simulink model "symbolTask"  (R2012b)
settings: Solver=FixedStepDiscrete  StartTime=0.0  StopTime=10.0  FixedStep=0.001  RelTol=1e-3
undefined symbols (not defined in the file): acquireMethods, autoplayMovementDuration, autoplayReactionTime, autoplayRotationDuration, autoplayRotationStart, centerOffset, clickPercentage, clickRefractoryPeriod, clickTargetColor, clickTargetHoverColor, cuedText, cuedTextLength, cumulativeDwell, cursorColorClick, cursorColorClosed, cursorColorOpen, cursorDiameter, cursorNeuralColor, cursorNonneuralColor, delayOrder, delayPeriodGainScale, displayObject, doHeadSpeedFail, drawNumbersOnTargets, dwellRefractoryPeriod, errorAssistAxis, errorAssistR, errorAssistTheta, expRandBinSize, expRandMax, expRandMin, expRandMu, eyeMode, failOnLiftoff, failurePenalty, falseClickFails, fingerPositionTolerance, fixedSeqMode, freePlayMode, gain, gloveBias, gloveLPDenominator, gloveLPNumerator, gloveNonlinearCorrection, gloveXCorrection, gloveYCorrection, gridEdges, gridTilesEachDim, headSpeedCap, holdDuration, holdTime, initialInput, initialLockout, initialState, inputType, keyboard, keyboardDims, keyPressedTime, lockFingerPosition, maxTaskTime ... (+103)
settings Model: Creator=gilja  LastModifiedBy=NPTL
settings SolverCC: EnableConcurrentExecution=on  ConcurrentTasks=on
settings DataIOCC: SaveOutput=off  SignalLogging=off  SaveTime=off
settings OptimizationCC: InlineParams=on  InlineInvariantSignals=on  EnhancedBackFolding=on  EfficientFloat2IntCast=on  SimCompilerOptimization=On
settings DebuggingCC: UnderspecifiedInitializationDetection=Simplified
settings HardwareCC: ProdIntDivRoundTo=Zero  ProdEndianess=LittleEndian  ProdHWDeviceType=Generic->32-bit x86 compatible
settings RTWCC: SystemTargetFile=xpctarget.tlc  TemplateMakefile=xpc_default_tmf  Description=xPC Target  ProcessScript=xpctarget_make_rtw_hook  RTWCompilerOptimization=On
settings CodeAppCC: MaxIdLength=62
settings xpcTargetCC: TargetFcnLib=ansi_tfl_table_tmw.mat  CodeReplacementLibrary=XPC_BLAS  ParMdlRefBuildCompliant=on  ConcurrentExecutionCompliant=on  CombineSignalStateStructs=off  GRTInterface=on  xPCTaskExecutionProfile=on  xPCRL32EventNumber=5000  xPCisDownloadable=off  xPCLoadParamSetFile=off  xPCConcurrentTasks=off  xPCEnableSFAnimation=off

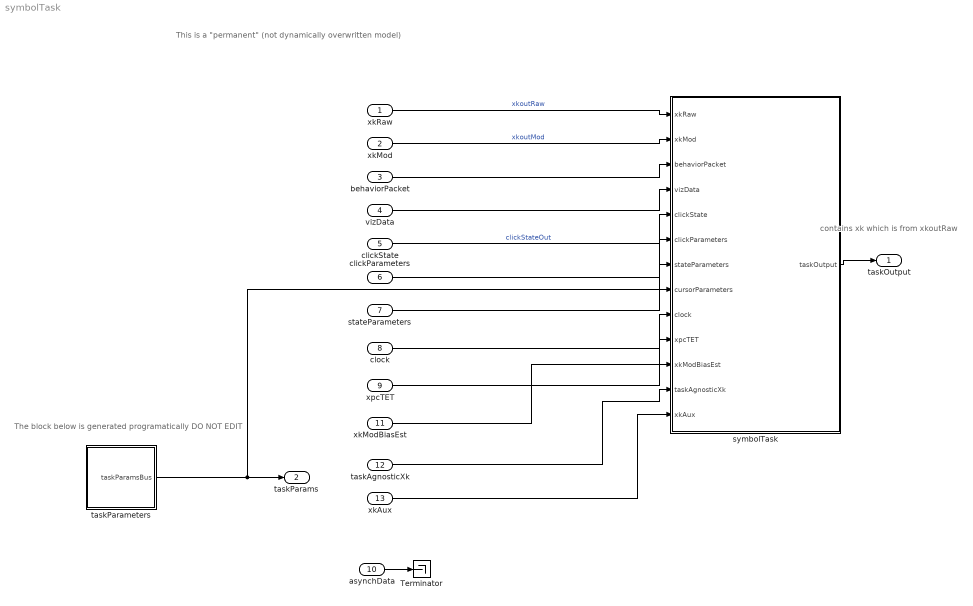
== system symbolTask ==
  note: contains xk which is
      | from xkoutRaw
  note: This is a "permanent" (not dynamically overwritten model)
  note: The block below is generated programatically
      | DO NOT EDIT
  xkRaw : Inport  OutDataTypeStr=double  PortDimensions=[double(xkConstants.NUM_STATE_DIMENSIONS),1]  SampleTime=[0.001,0]
  xkMod : Inport  Port=2  OutDataTypeStr=double  PortDimensions=[double(xkConstants.NUM_STATE_DIMENSIONS),1]  SampleTime=[0.001,0]
  behaviorPacket : Inport  Port=3  OutDataTypeStr=Bus: behaviorPacketBus  SampleTime=[0.001,0]
  vizData : Inport  Port=4  OutDataTypeStr=Bus: peripheralData  SampleTime=[0.001,0]
  clickState : Inport  Port=5  OutDataTypeStr=uint16  PortDimensions=1  SampleTime=[0.001,0]
  clickParameters : Inport  Port=6  OutDataTypeStr=Bus: clickParametersBus  SampleTime=[0.001,0]
  stateParameters : Inport  Port=7  OutDataTypeStr=Bus: stateParams  SampleTime=[0.001,0]
  clock : Inport  Port=8  OutDataTypeStr=uint32  PortDimensions=1  SampleTime=[0.001,0]
  xpcTET : Inport  Port=9  OutDataTypeStr=double  PortDimensions=1  SampleTime=[0.001,0]
  asynchData : Inport  Port=10  OutDataTypeStr=Bus: peripheralData  SampleTime=[0.001,0]
  xkModBiasEst : Inport  Port=11  OutDataTypeStr=double  PortDimensions=[double(xkConstants.NUM_STATE_DIMENSIONS),1]  SampleTime=[0.001,0]
  taskAgnosticXk : Inport  Port=12  OutDataTypeStr=double  PortDimensions=[double(xkConstants.NUM_STATE_DIMENSIONS),1]  SampleTime=[0.001,0]
  xkAux : Inport  Port=13  OutDataTypeStr=double  PortDimensions=[double(xkConstants.NUM_STATE_DIMENSIONS),1]  SampleTime=[0.001,0]
  Terminator : Terminator
  symbolTask : MATLAB Function  TreatAsAtomicUnit=on
  taskParameters : Subsystem
  taskOutput : Outport  OutDataTypeStr=Bus: taskOutput  PortDimensions=1  SampleTime=[0.001,0]  BusOutputAsStruct=on
  taskParams : Outport  Port=2  OutDataTypeStr=Bus: taskParamsBus  SampleTime=[0.001,0]
  wires:
  xkRaw/1 -> symbolTask/1(xkRaw)  "xkoutRaw"
  behaviorPacket/1 -> symbolTask/3(behaviorPacket)
  vizData/1 -> symbolTask/4(vizData)
  clickState/1 -> symbolTask/5(clickState)  "clickStateOut"
  clickParameters/1 -> symbolTask/6(clickParameters)
  clock/1 -> symbolTask/9(clock)
  xpcTET/1 -> symbolTask/10(xpcTET)
  stateParameters/1 -> symbolTask/7(stateParameters)
  taskParameters/1(taskParamsBus) -> taskParams/1, symbolTask/8(cursorParameters)
  symbolTask/1(taskOutput) -> taskOutput/1
  asynchData/1 -> Terminator/1
  xkMod/1 -> symbolTask/2(xkMod)  "xkoutMod"
  xkModBiasEst/1 -> symbolTask/11(xkModBiasEst)
  taskAgnosticXk/1 -> symbolTask/12(taskAgnosticXk)
  xkAux/1 -> symbolTask/13(xkAux)

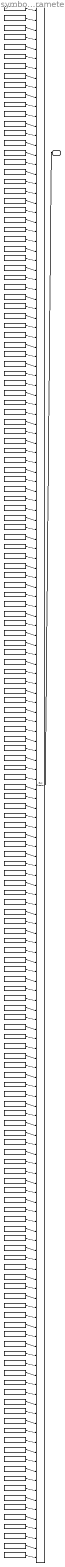
== system symbolTask/taskParameters ==
  BusOutput : BusCreator  Inputs=targetDiameter,maxTaskTime,holdTime,trialTimeout,numTrials,randomSeed,expRandMu,expRandMin,expRandMax,expRandBinSize,taskType,targetInds,numTargets,gain,failurePenalty,cursorDiameter,inputType,gloveBias,useRandomDelay,mouseOffset,workspaceX,workspaceY,workspaceZ,workspaceR,workspaceR2,showScores,trialsPerScore,cursorColorClick,recenterOnFail,recenterOnSuccess,recenterDelay,initialInput,clickPercentage,lockFingerPosition,fingerPositionTolerance,failOnLiftoff,errorAssistR,errorAssistTheta,errorAssistAxis,useGloveLPF,gloveLPNumerator,gloveLPDenominator,gloveNonlinearCorrection,gloveYCorrection,gloveXCorrection,useMouseLPF,soundOnFail,soundOnGo,soundOnSuccess,soundOnOverTarget,mouseLPNumerator,mouseLPDenominator,stopOffTarget,stopOnClick,outputType,xk2HorizontalPos,xk2HorizontalVel,xk2VerticalPos,xk2VerticalVel,xk2DepthPos,xk2DepthVel,xk2RotatePos,xk2RotateVel,xk2Rotate2Pos,xk2Rotate2Vel,gridEdges,gridTilesEachDim,selectionRefractoryMS,autoplayReactionTime,autoplayMovementDuration,powerGain,powerGainUnityCrossing,targetRotDiameter,autoplayRotationStart,autoplayRotationDuration,randomTaskTargetDiameters,randomTaskTargetRotDiameters,randomTaskBoundaries,numDisplayDims,cursorColorOpen,cursorColorClosed,showXYZaura,displayObject,preTrialLength,targetDiameters,numTargetDiameters,minTargetDistance,targetDelay,targetSpaceX,targetSpaceY,clickTargetColor,clickTargetHoverColor,falseClickFails,splitDimensions,vmrTheta,doHeadSpeedFail,headSpeedCap,eyeMode,speedTaskMode,delayPeriodGainScale,wiaMode,showWiaText,freePlayMode,drawNumbersOnTargets,xkRawSpeedCap,movementDuration,holdDuration,restDuration,returnDuration,repsPerBlock,whichMovements,movementOrder,delayOrder,clickRefractoryPeriod,xpcVelocityOutputPeriodMS,outputVelocityScaling,screenUpdateRate,targetDevice,playSpokenCues,numTargetsInSeq,targetSeq,seqReadyTime,seqRehearseTime,rotateSeqCues,numRepsPerSeq,rehearsalOrder,rehearsalTimes,pathMode,memorizeMode,fixedSeqMode,sequenceMatrix,keyboard,resetDisplay,cursorNeuralColor,cursorNonneuralColor,centerOffset,scoreTime,cuedTextLength,cuedText,keyboardDims,recenterFullscreen,soundOnError,acquireMethods,cumulativeDwell,showBackspace,showStartStop,showTargetText,showTypedText,showCueOnTarget,showCueOffTarget,recenterOffset,dwellRefractoryPeriod,keyPressedTime,initialLockout,initialState,symbolMoveTimeOne,symbolRehearseTime,symbolGetReadyTime,symbolMoveTimeTwo,symbolVMRMode,symbolVMRRot,pc1MouseInControlMode  OutDataTypeStr=Bus: taskParamsBus
  acquireMethods : Constant  Value=acquireMethods
  autoplayMovementDuration : Constant  Value=autoplayMovementDuration
  autoplayReactionTime : Constant  Value=autoplayReactionTime
  autoplayRotationDuration : Constant  Value=autoplayRotationDuration
  autoplayRotationStart : Constant  Value=autoplayRotationStart
  centerOffset : Constant  Value=centerOffset
  clickPercentage : Constant  Value=clickPercentage
  clickRefractoryPeriod : Constant  Value=clickRefractoryPeriod
  clickTargetColor : Constant  Value=clickTargetColor
  clickTargetHoverColor : Constant  Value=clickTargetHoverColor
  cuedText : Constant  Value=cuedText
  cuedTextLength : Constant  Value=cuedTextLength
  cumulativeDwell : Constant  Value=cumulativeDwell
  cursorColorClick : Constant  Value=cursorColorClick
  cursorColorClosed : Constant  Value=cursorColorClosed
  cursorColorOpen : Constant  Value=cursorColorOpen
  cursorDiameter : Constant  Value=cursorDiameter
  cursorNeuralColor : Constant  Value=cursorNeuralColor
  cursorNonneuralColor : Constant  Value=cursorNonneuralColor
  delayOrder : Constant  Value=delayOrder
  delayPeriodGainScale : Constant  Value=delayPeriodGainScale
  displayObject : Constant  Value=displayObject
  doHeadSpeedFail : Constant  Value=doHeadSpeedFail
  drawNumbersOnTargets : Constant  Value=drawNumbersOnTargets
  dwellRefractoryPeriod : Constant  Value=dwellRefractoryPeriod
  errorAssistAxis : Constant  Value=errorAssistAxis
  errorAssistR : Constant  Value=errorAssistR
  errorAssistTheta : Constant  Value=errorAssistTheta
  expRandBinSize : Constant  Value=expRandBinSize
  expRandMax : Constant  Value=expRandMax
  expRandMin : Constant  Value=expRandMin
  expRandMu : Constant  Value=expRandMu
  eyeMode : Constant  Value=eyeMode
  failOnLiftoff : Constant  Value=failOnLiftoff
  failurePenalty : Constant  Value=failurePenalty
  falseClickFails : Constant  Value=falseClickFails
  fingerPositionTolerance : Constant  Value=fingerPositionTolerance
  fixedSeqMode : Constant  Value=fixedSeqMode
  freePlayMode : Constant  Value=freePlayMode
  gain : Constant  Value=gain
  gloveBias : Constant  Value=gloveBias
  gloveLPDenominator : Constant  Value=gloveLPDenominator
  gloveLPNumerator : Constant  Value=gloveLPNumerator
  gloveNonlinearCorrection : Constant  Value=gloveNonlinearCorrection
  gloveXCorrection : Constant  Value=gloveXCorrection
  gloveYCorrection : Constant  Value=gloveYCorrection
  gridEdges : Constant  Value=gridEdges
  gridTilesEachDim : Constant  Value=gridTilesEachDim
  headSpeedCap : Constant  Value=headSpeedCap
  holdDuration : Constant  Value=holdDuration
  holdTime : Constant  Value=holdTime
  initialInput : Constant  Value=initialInput
  initialLockout : Constant  Value=initialLockout
  initialState : Constant  Value=initialState
  inputType : Constant  Value=inputType
  keyPressedTime : Constant  Value=keyPressedTime
  keyboard : Constant  Value=keyboard
  keyboardDims : Constant  Value=keyboardDims
  lockFingerPosition : Constant  Value=lockFingerPosition
  maxTaskTime : Constant  Value=maxTaskTime
  memorizeMode : Constant  Value=memorizeMode
  minTargetDistance : Constant  Value=minTargetDistance
  mouseLPDenominator : Constant  Value=mouseLPDenominator
  mouseLPNumerator : Constant  Value=mouseLPNumerator
  mouseOffset : Constant  Value=mouseOffset
  movementDuration : Constant  Value=movementDuration
  movementOrder : Constant  Value=movementOrder
  numDisplayDims : Constant  Value=numDisplayDims
  numRepsPerSeq : Constant  Value=numRepsPerSeq
  numTargetDiameters : Constant  Value=numTargetDiameters
  numTargets : Constant  Value=numTargets
  numTargetsInSeq : Constant  Value=numTargetsInSeq
  numTrials : Constant  Value=numTrials
  outputType : Constant  Value=outputType
  outputVelocityScaling : Constant  Value=outputVelocityScaling
  pathMode : Constant  Value=pathMode
  pc1MouseInControlMode : Constant  Value=pc1MouseInControlMode
  playSpokenCues : Constant  Value=playSpokenCues
  powerGain : Constant  Value=powerGain
  powerGainUnityCrossing : Constant  Value=powerGainUnityCrossing
  preTrialLength : Constant  Value=preTrialLength
  randomSeed : Constant  Value=randomSeed
  randomTaskBoundaries : Constant  Value=randomTaskBoundaries
  randomTaskTargetDiameters : Constant  Value=randomTaskTargetDiameters
  randomTaskTargetRotDiameters : Constant  Value=randomTaskTargetRotDiameters
  recenterDelay : Constant  Value=recenterDelay
  recenterFullscreen : Constant  Value=recenterFullscreen
  recenterOffset : Constant  Value=recenterOffset
  recenterOnFail : Constant  Value=recenterOnFail
  recenterOnSuccess : Constant  Value=recenterOnSuccess
  rehearsalOrder : Constant  Value=rehearsalOrder
  rehearsalTimes : Constant  Value=rehearsalTimes
  repsPerBlock : Constant  Value=repsPerBlock
  resetDisplay : Constant  Value=resetDisplay
  restDuration : Constant  Value=restDuration
  returnDuration : Constant  Value=returnDuration
  rotateSeqCues : Constant  Value=rotateSeqCues
  scoreTime : Constant  Value=scoreTime
  screenUpdateRate : Constant  Value=screenUpdateRate
  selectionRefractoryMS : Constant  Value=selectionRefractoryMS
  seqReadyTime : Constant  Value=seqReadyTime
  seqRehearseTime : Constant  Value=seqRehearseTime
  sequenceMatrix : Constant  Value=sequenceMatrix
  showBackspace : Constant  Value=showBackspace
  showCueOffTarget : Constant  Value=showCueOffTarget
  showCueOnTarget : Constant  Value=showCueOnTarget
  showScores : Constant  Value=showScores
  showStartStop : Constant  Value=showStartStop
  showTargetText : Constant  Value=showTargetText
  showTypedText : Constant  Value=showTypedText
  showWiaText : Constant  Value=showWiaText
  showXYZaura : Constant  Value=showXYZaura
  soundOnError : Constant  Value=soundOnError
  soundOnFail : Constant  Value=soundOnFail
  soundOnGo : Constant  Value=soundOnGo
  soundOnOverTarget : Constant  Value=soundOnOverTarget
  soundOnSuccess : Constant  Value=soundOnSuccess
  speedTaskMode : Constant  Value=speedTaskMode
  splitDimensions : Constant  Value=splitDimensions
  stopOffTarget : Constant  Value=stopOffTarget
  stopOnClick : Constant  Value=stopOnClick
  symbolGetReadyTime : Constant  Value=symbolGetReadyTime
  symbolMoveTimeOne : Constant  Value=symbolMoveTimeOne
  symbolMoveTimeTwo : Constant  Value=symbolMoveTimeTwo
  symbolRehearseTime : Constant  Value=symbolRehearseTime
  symbolVMRMode : Constant  Value=symbolVMRMode
  symbolVMRRot : Constant  Value=symbolVMRRot
  targetDelay : Constant  Value=targetDelay
  targetDevice : Constant  Value=targetDevice
  targetDiameter : Constant  Value=targetDiameter
  targetDiameters : Constant  Value=targetDiameters
  targetInds : Constant  Value=targetInds
  targetRotDiameter : Constant  Value=targetRotDiameter
  targetSeq : Constant  Value=targetSeq
  targetSpaceX : Constant  Value=targetSpaceX
  targetSpaceY : Constant  Value=targetSpaceY
  taskType : Constant  Value=taskType
  trialTimeout : Constant  Value=trialTimeout
  trialsPerScore : Constant  Value=trialsPerScore
  useGloveLPF : Constant  Value=useGloveLPF
  useMouseLPF : Constant  Value=useMouseLPF
  useRandomDelay : Constant  Value=useRandomDelay
  vmrTheta : Constant  Value=vmrTheta
  whichMovements : Constant  Value=whichMovements
  wiaMode : Constant  Value=wiaMode
  workspaceR : Constant  Value=workspaceR
  workspaceR2 : Constant  Value=workspaceR2
  workspaceX : Constant  Value=workspaceX
  workspaceY : Constant  Value=workspaceY
  workspaceZ : Constant  Value=workspaceZ
  xk2DepthPos : Constant  Value=xk2DepthPos
  xk2DepthVel : Constant  Value=xk2DepthVel
  xk2HorizontalPos : Constant  Value=xk2HorizontalPos
  xk2HorizontalVel : Constant  Value=xk2HorizontalVel
  xk2Rotate2Pos : Constant  Value=xk2Rotate2Pos
  xk2Rotate2Vel : Constant  Value=xk2Rotate2Vel
  xk2RotatePos : Constant  Value=xk2RotatePos
  xk2RotateVel : Constant  Value=xk2RotateVel
  xk2VerticalPos : Constant  Value=xk2VerticalPos
  xk2VerticalVel : Constant  Value=xk2VerticalVel
  xkRawSpeedCap : Constant  Value=xkRawSpeedCap
  xpcVelocityOutputPeriodMS : Constant  Value=xpcVelocityOutputPeriodMS
  taskParamsBus : Outport
  wires:
  targetDiameter/1 -> BusOutput/1  "targetDiameter"
  maxTaskTime/1 -> BusOutput/2  "maxTaskTime"
  holdTime/1 -> BusOutput/3  "holdTime"
  trialTimeout/1 -> BusOutput/4  "trialTimeout"
  numTrials/1 -> BusOutput/5  "numTrials"
  randomSeed/1 -> BusOutput/6  "randomSeed"
  expRandMu/1 -> BusOutput/7  "expRandMu"
  expRandMin/1 -> BusOutput/8  "expRandMin"
  expRandMax/1 -> BusOutput/9  "expRandMax"
  expRandBinSize/1 -> BusOutput/10  "expRandBinSize"
  taskType/1 -> BusOutput/11  "taskType"
  targetInds/1 -> BusOutput/12  "targetInds"
  numTargets/1 -> BusOutput/13  "numTargets"
  gain/1 -> BusOutput/14  "gain"
  failurePenalty/1 -> BusOutput/15  "failurePenalty"
  cursorDiameter/1 -> BusOutput/16  "cursorDiameter"
  inputType/1 -> BusOutput/17  "inputType"
  gloveBias/1 -> BusOutput/18  "gloveBias"
  useRandomDelay/1 -> BusOutput/19  "useRandomDelay"
  mouseOffset/1 -> BusOutput/20  "mouseOffset"
  workspaceX/1 -> BusOutput/21  "workspaceX"
  workspaceY/1 -> BusOutput/22  "workspaceY"
  workspaceZ/1 -> BusOutput/23  "workspaceZ"
  workspaceR/1 -> BusOutput/24  "workspaceR"
  workspaceR2/1 -> BusOutput/25  "workspaceR2"
  showScores/1 -> BusOutput/26  "showScores"
  trialsPerScore/1 -> BusOutput/27  "trialsPerScore"
  cursorColorClick/1 -> BusOutput/28  "cursorColorClick"
  recenterOnFail/1 -> BusOutput/29  "recenterOnFail"
  recenterOnSuccess/1 -> BusOutput/30  "recenterOnSuccess"
  recenterDelay/1 -> BusOutput/31  "recenterDelay"
  initialInput/1 -> BusOutput/32  "initialInput"
  clickPercentage/1 -> BusOutput/33  "clickPercentage"
  lockFingerPosition/1 -> BusOutput/34  "lockFingerPosition"
  fingerPositionTolerance/1 -> BusOutput/35  "fingerPositionTolerance"
  failOnLiftoff/1 -> BusOutput/36  "failOnLiftoff"
  errorAssistR/1 -> BusOutput/37  "errorAssistR"
  errorAssistTheta/1 -> BusOutput/38  "errorAssistTheta"
  errorAssistAxis/1 -> BusOutput/39  "errorAssistAxis"
  useGloveLPF/1 -> BusOutput/40  "useGloveLPF"
  gloveLPNumerator/1 -> BusOutput/41  "gloveLPNumerator"
  gloveLPDenominator/1 -> BusOutput/42  "gloveLPDenominator"
  gloveNonlinearCorrection/1 -> BusOutput/43  "gloveNonlinearCorrection"
  gloveYCorrection/1 -> BusOutput/44  "gloveYCorrection"
  gloveXCorrection/1 -> BusOutput/45  "gloveXCorrection"
  useMouseLPF/1 -> BusOutput/46  "useMouseLPF"
  soundOnFail/1 -> BusOutput/47  "soundOnFail"
  soundOnGo/1 -> BusOutput/48  "soundOnGo"
  soundOnSuccess/1 -> BusOutput/49  "soundOnSuccess"
  soundOnOverTarget/1 -> BusOutput/50  "soundOnOverTarget"
  mouseLPNumerator/1 -> BusOutput/51  "mouseLPNumerator"
  mouseLPDenominator/1 -> BusOutput/52  "mouseLPDenominator"
  stopOffTarget/1 -> BusOutput/53  "stopOffTarget"
  stopOnClick/1 -> BusOutput/54  "stopOnClick"
  outputType/1 -> BusOutput/55  "outputType"
  xk2HorizontalPos/1 -> BusOutput/56  "xk2HorizontalPos"
  xk2HorizontalVel/1 -> BusOutput/57  "xk2HorizontalVel"
  xk2VerticalPos/1 -> BusOutput/58  "xk2VerticalPos"
  xk2VerticalVel/1 -> BusOutput/59  "xk2VerticalVel"
  xk2DepthPos/1 -> BusOutput/60  "xk2DepthPos"
  xk2DepthVel/1 -> BusOutput/61  "xk2DepthVel"
  xk2RotatePos/1 -> BusOutput/62  "xk2RotatePos"
  xk2RotateVel/1 -> BusOutput/63  "xk2RotateVel"
  xk2Rotate2Pos/1 -> BusOutput/64  "xk2Rotate2Pos"
  xk2Rotate2Vel/1 -> BusOutput/65  "xk2Rotate2Vel"
  gridEdges/1 -> BusOutput/66  "gridEdges"
  gridTilesEachDim/1 -> BusOutput/67  "gridTilesEachDim"
  selectionRefractoryMS/1 -> BusOutput/68  "selectionRefractoryMS"
  autoplayReactionTime/1 -> BusOutput/69  "autoplayReactionTime"
  autoplayMovementDuration/1 -> BusOutput/70  "autoplayMovementDuration"
  powerGain/1 -> BusOutput/71  "powerGain"
  powerGainUnityCrossing/1 -> BusOutput/72  "powerGainUnityCrossing"
  targetRotDiameter/1 -> BusOutput/73  "targetRotDiameter"
  autoplayRotationStart/1 -> BusOutput/74  "autoplayRotationStart"
  autoplayRotationDuration/1 -> BusOutput/75  "autoplayRotationDuration"
  randomTaskTargetDiameters/1 -> BusOutput/76  "randomTaskTargetDiameters"
  randomTaskTargetRotDiameters/1 -> BusOutput/77  "randomTaskTargetRotDiameters"
  randomTaskBoundaries/1 -> BusOutput/78  "randomTaskBoundaries"
  numDisplayDims/1 -> BusOutput/79  "numDisplayDims"
  cursorColorOpen/1 -> BusOutput/80  "cursorColorOpen"
  cursorColorClosed/1 -> BusOutput/81  "cursorColorClosed"
  showXYZaura/1 -> BusOutput/82  "showXYZaura"
  displayObject/1 -> BusOutput/83  "displayObject"
  preTrialLength/1 -> BusOutput/84  "preTrialLength"
  targetDiameters/1 -> BusOutput/85  "targetDiameters"
  numTargetDiameters/1 -> BusOutput/86  "numTargetDiameters"
  minTargetDistance/1 -> BusOutput/87  "minTargetDistance"
  targetDelay/1 -> BusOutput/88  "targetDelay"
  targetSpaceX/1 -> BusOutput/89  "targetSpaceX"
  targetSpaceY/1 -> BusOutput/90  "targetSpaceY"
  clickTargetColor/1 -> BusOutput/91  "clickTargetColor"
  clickTargetHoverColor/1 -> BusOutput/92  "clickTargetHoverColor"
  falseClickFails/1 -> BusOutput/93  "falseClickFails"
  splitDimensions/1 -> BusOutput/94  "splitDimensions"
  vmrTheta/1 -> BusOutput/95  "vmrTheta"
  doHeadSpeedFail/1 -> BusOutput/96  "doHeadSpeedFail"
  headSpeedCap/1 -> BusOutput/97  "headSpeedCap"
  eyeMode/1 -> BusOutput/98  "eyeMode"
  speedTaskMode/1 -> BusOutput/99  "speedTaskMode"
  delayPeriodGainScale/1 -> BusOutput/100  "delayPeriodGainScale"
  wiaMode/1 -> BusOutput/101  "wiaMode"
  showWiaText/1 -> BusOutput/102  "showWiaText"
  freePlayMode/1 -> BusOutput/103  "freePlayMode"
  drawNumbersOnTargets/1 -> BusOutput/104  "drawNumbersOnTargets"
  xkRawSpeedCap/1 -> BusOutput/105  "xkRawSpeedCap"
  movementDuration/1 -> BusOutput/106  "movementDuration"
  holdDuration/1 -> BusOutput/107  "holdDuration"
  restDuration/1 -> BusOutput/108  "restDuration"
  returnDuration/1 -> BusOutput/109  "returnDuration"
  repsPerBlock/1 -> BusOutput/110  "repsPerBlock"
  whichMovements/1 -> BusOutput/111  "whichMovements"
  movementOrder/1 -> BusOutput/112  "movementOrder"
  delayOrder/1 -> BusOutput/113  "delayOrder"
  clickRefractoryPeriod/1 -> BusOutput/114  "clickRefractoryPeriod"
  xpcVelocityOutputPeriodMS/1 -> BusOutput/115  "xpcVelocityOutputPeriodMS"
  outputVelocityScaling/1 -> BusOutput/116  "outputVelocityScaling"
  screenUpdateRate/1 -> BusOutput/117  "screenUpdateRate"
  targetDevice/1 -> BusOutput/118  "targetDevice"
  playSpokenCues/1 -> BusOutput/119  "playSpokenCues"
  numTargetsInSeq/1 -> BusOutput/120  "numTargetsInSeq"
  targetSeq/1 -> BusOutput/121  "targetSeq"
  seqReadyTime/1 -> BusOutput/122  "seqReadyTime"
  seqRehearseTime/1 -> BusOutput/123  "seqRehearseTime"
  rotateSeqCues/1 -> BusOutput/124  "rotateSeqCues"
  numRepsPerSeq/1 -> BusOutput/125  "numRepsPerSeq"
  rehearsalOrder/1 -> BusOutput/126  "rehearsalOrder"
  rehearsalTimes/1 -> BusOutput/127  "rehearsalTimes"
  pathMode/1 -> BusOutput/128  "pathMode"
  memorizeMode/1 -> BusOutput/129  "memorizeMode"
  fixedSeqMode/1 -> BusOutput/130  "fixedSeqMode"
  sequenceMatrix/1 -> BusOutput/131  "sequenceMatrix"
  keyboard/1 -> BusOutput/132  "keyboard"
  resetDisplay/1 -> BusOutput/133  "resetDisplay"
  cursorNeuralColor/1 -> BusOutput/134  "cursorNeuralColor"
  cursorNonneuralColor/1 -> BusOutput/135  "cursorNonneuralColor"
  centerOffset/1 -> BusOutput/136  "centerOffset"
  scoreTime/1 -> BusOutput/137  "scoreTime"
  cuedTextLength/1 -> BusOutput/138  "cuedTextLength"
  cuedText/1 -> BusOutput/139  "cuedText"
  keyboardDims/1 -> BusOutput/140  "keyboardDims"
  recenterFullscreen/1 -> BusOutput/141  "recenterFullscreen"
  soundOnError/1 -> BusOutput/142  "soundOnError"
  acquireMethods/1 -> BusOutput/143  "acquireMethods"
  cumulativeDwell/1 -> BusOutput/144  "cumulativeDwell"
  showBackspace/1 -> BusOutput/145  "showBackspace"
  showStartStop/1 -> BusOutput/146  "showStartStop"
  showTargetText/1 -> BusOutput/147  "showTargetText"
  showTypedText/1 -> BusOutput/148  "showTypedText"
  showCueOnTarget/1 -> BusOutput/149  "showCueOnTarget"
  showCueOffTarget/1 -> BusOutput/150  "showCueOffTarget"
  recenterOffset/1 -> BusOutput/151  "recenterOffset"
  dwellRefractoryPeriod/1 -> BusOutput/152  "dwellRefractoryPeriod"
  keyPressedTime/1 -> BusOutput/153  "keyPressedTime"
  initialLockout/1 -> BusOutput/154  "initialLockout"
  initialState/1 -> BusOutput/155  "initialState"
  symbolMoveTimeOne/1 -> BusOutput/156  "symbolMoveTimeOne"
  symbolRehearseTime/1 -> BusOutput/157  "symbolRehearseTime"
  symbolGetReadyTime/1 -> BusOutput/158  "symbolGetReadyTime"
  symbolMoveTimeTwo/1 -> BusOutput/159  "symbolMoveTimeTwo"
  symbolVMRMode/1 -> BusOutput/160  "symbolVMRMode"
  symbolVMRRot/1 -> BusOutput/161  "symbolVMRRot"
  pc1MouseInControlMode/1 -> BusOutput/162  "pc1MouseInControlMode"
  BusOutput/1 -> taskParamsBus/1

== matlab function symbolTask/symbolTask ==
  data: xkRaw input double size=[double(xkConstants.NUM_STATE_DIMENSIONS) 1]; xkMod input; behaviorPacket input Bus: behaviorPacketBus size=1; vizData input Bus: peripheralData; clickState input; clickParameters input; taskOutput output Bus: taskOutput; stateParameters input Bus: stateParams size=1; cursorParameters input Bus: taskParamsBus; clock input; xpcTET input; xkModBiasEst input; taskAgnosticXk input; xkAux input
function taskOutput  = symbolTask(xkRaw, xkMod, behaviorPacket, vizData, clickState, clickParameters, ...
    stateParameters, cursorParameters, clock, xpcTET, xkModBiasEst, taskAgnosticXk, xkAux)

%#codegen
behaviorRequestClock = behaviorPacket.xpcRequestClock;
peripheralTimestamp = behaviorPacket.peripheralTimestamp(1:16);

%% CONSTANTS
TASK_NAME = 'symbol';
VERSION_ID = single(1.0);

%% INITIALIZE CURSOR TASK OUTPUT
fileLoggerData.data = uint8(zeros(1,1400));
fileLoggerData.dataLen = uint16(0);
fileLoggerData.fileName = uint8(zeros(1,20));
fileLoggerData.send = false;

fileLoggerFormat.format = uint8(zeros(1,1400));
fileLoggerFormat.formatLen = uint16(0);
fileLoggerFormat.fileName = uint8(zeros(1,20));

fileLoggerFormatAndData.format = fileLoggerFormat;
fileLoggerFormatAndData.data = fileLoggerData;

taskOutput.flushFiles = false;
taskOutput.sendFormat = false;
taskOutput.taskDetails = fileLoggerFormat;
taskOutput.discrete = fileLoggerFormatAndData;
taskOutput.continuous = fileLoggerFormatAndData;
taskOutput.screen = fileLoggerFormatAndData;
taskOutput.sound = fileLoggerFormatAndData;
taskOutput.asynch = fileLoggerFormatAndData;
taskOutput.ttl = double(0);
taskOutput.xk = xkRaw;
taskOutput.inputType = cursorParameters.inputType;
taskOutput.currentTarget = single(zeros([double(xkConstants.NUM_TARGET_DIMENSIONS) 1]));
taskOutput.state = uint16(SequenceStates.STATE_MOVE);
taskOutput.paused = false;
taskOutput.allowStop = true;
taskOutput.resetHMM = true;

%% TASK DETAILS PACKET
taskOutput.taskDetails = packFileLoggerTaskDetails(TASK_NAME, VERSION_ID, ...
    'STATE_INIT', uint8(SymbolStates.STATE_INIT), ...
    'STATE_MOVE_ONE', uint8(SymbolStates.STATE_MOVE_ONE),...
    'STATE_MOVE_TWO', uint8(SymbolStates.STATE_MOVE_TWO),...
    'STATE_REHEARSE', uint8(SymbolStates.STATE_REHEARSE), ...
    'STATE_READY', uint8(SymbolStates.STATE_READY),...
    'INPUT_TYPE_DECODE_V', uint8(cursorConstants.INPUT_TYPE_DECODE_V),...
    'INPUT_TYPE_HEAD_MOUSE', uint8(cursorConstants.INPUT_TYPE_HEAD_MOUSE) ...
);

%% DEFINE PERSISTENTS
persistent holdTimer readyTimer rehearseTimer moveTimer;

persistent numTargetsAcquired;
persistent summedAcquireTime;
persistent state;
persistent currentTarg;
persistent allTargPos;
persistent lastTarget;

persistent rehearseSet;
persistent currentSymbolSet;
persistent allSymbols;
persistent currentSymbolIdx;

persistent setMoveTimeOne;
persistent setRehearseTime;
persistent setGetReadyTime;
persistent setMoveTimeTwo;

persistent recenteringState;

persistent lastSoundTime;
persistent lastSoundState;
persistent cursorColors;
persistent vizPacket;
persistent showFailedTarg;
persistent pastPause;
persistent targetSeq;
persistent targetSeqIdx;

persistent prevTargAcquireTime;
persistent lastAcquireTime;
persistent numSetsComplete;
persistent writeFailedTarg;
persistent prevHeadPos;
persistent filteredHeadSpeed;
persistent lastHeadSpeedFail;

%% INITIALIZE PERSISTENTS
NUM_TARG = uint16(8);
if(isempty(holdTimer))
    holdTimer = uint16(0);
    readyTimer = uint32(0);
    rehearseTimer = uint32(0);
    moveTimer = uint32(0);

    numTargetsAcquired = uint16(0);
    summedAcquireTime = uint32(0);
    state = uint8(SymbolStates.STATE_INIT);
    currentTarg = uint16(0);
    lastTarget = uint16(0);
    allTargPos = cursorParameters.targetInds;
    prevHeadPos = single(zeros(2,1));
    filteredHeadSpeed = single(0);
    lastHeadSpeedFail = uint32(0);
    
    rehearseSet = false;
    allSymbols = uint16(zeros(100,1));
    allSymbols(1:100) = 1:100;
    currentSymbolSet = uint16(zeros(NUM_TARG,1));
    currentSymbolIdx = uint16(1);
    numSetsComplete = uint16(0);

    setMoveTimeOne = cursorParameters.symbolMoveTimeOne;
    setRehearseTime = cursorParameters.symbolRehearseTime;
    setGetReadyTime = cursorParameters.symbolGetReadyTime;
    setMoveTimeTwo = cursorParameters.symbolMoveTimeTwo;

    lastSoundTime = clock;
    lastSoundState = uint8(SequenceStates.SOUND_STATE_IDLE);

    cursorColors = double(zeros([3 2]));
    vizPacket = initVizPacket();
    showFailedTarg = false;
    pastPause = false;
    
    targetSeq = uint16(zeros(1,NUM_TARG));
    targetSeqIdx = uint16(1);
    
    recenteringState = true;
    lastAcquireTime = clock;
    prevTargAcquireTime = clock;
    
    writeFailedTarg = false;
end
inputType = cursorParameters.inputType;

%% some initialization
outputType = cursorParameters.outputType; % determines what graphics engine will render this task.

writeDiscreteData = false;
writeContinuousData = true;
writeToDiscreteTarg = uint16(0);

if(vizData.receive && (vizData.dataLen > 0 ))
    vizPacket = parseVizPacket(vizData.data);
end

xk2HorizontalPos = uint8( cursorParameters.xk2HorizontalPos );
xk2VerticalPos = uint8( cursorParameters.xk2VerticalPos );
xk2HorizontalVel = uint8( cursorParameters.xk2HorizontalVel );
xk2VerticalVel = uint8( cursorParameters.xk2VerticalVel );

effectorPosInds = [xk2HorizontalPos,xk2VerticalPos];
effectorVelInds = [xk2HorizontalVel,xk2VerticalVel];

effectorPos = xkMod(effectorPosInds);
effectorVel = xkMod(effectorVelInds);

if cursorParameters.pc1MouseInControlMode
    effectorPos(1) = behaviorPacket.pc1MousePos(1)*1080;
    effectorPos(2) = -behaviorPacket.pc1MousePos(2)*1080;
else
    effectorPos(1) = behaviorPacket.windowsMousePosition(1)*1080;
    effectorPos(2) = -behaviorPacket.windowsMousePosition(2)*1080;
end

INIT_TIME = uint32(2000);
pauseToggled = (pastPause==true) && (stateParameters.pause==false);
pauseTriggered = stateParameters.pause;
pastPause = stateParameters.pause;

if(clock < INIT_TIME)
    state = uint8(SymbolStates.STATE_INIT);
    pauseTriggered = true;
elseif (state == uint8(SymbolStates.STATE_INIT)) && pauseToggled
    targetSeq = uint16(randperm(NUM_TARG));
    targetSeqIdx = uint16(1);
    allTargPos = cursorParameters.targetInds;
    currentTarg = targetSeq(targetSeqIdx);
    
    shuffIdx = randperm(100);
    allSymbols = allSymbols(shuffIdx);

    currentSymbolIdx = uint16(1);
    readyTimer = setGetReadyTime;
    state = uint8(SymbolStates.STATE_READY);
end

setMoveTimeOne = cursorParameters.symbolMoveTimeOne;
setRehearseTime = cursorParameters.symbolRehearseTime;
setGetReadyTime = cursorParameters.symbolGetReadyTime;
setMoveTimeTwo = cursorParameters.symbolMoveTimeTwo;

%%
%continuously affect state of RNG so we get somewhat random numbers from
%run to run
junkVal = rand(1,1);

%% default colors
cursorColors(1:end,1) = [255; 255; 255;];

%%
%estimate movement speed
headSpeedAlpha = single(0.96);
headSpeed = 1000*sqrt(sum((behaviorPacket.windowsMousePosition - prevHeadPos).^2));
filteredHeadSpeed = headSpeedAlpha*filteredHeadSpeed + (1-headSpeedAlpha)*headSpeed;
prevHeadPos = behaviorPacket.windowsMousePosition;

%%
%manage rehearsal, get ready, move states
countdownDisplayTimer = uint32(0);
if state == uint8(SymbolStates.STATE_READY)
    readyTimer = readyTimer - 1;
    countdownDisplayTimer = readyTimer;
    if readyTimer<=0
        %new set of symbols      
        %newIdx = currentSymbolIdx:(currentSymbolIdx+NUM_TARG-1);
        %currentSymbolSet = allSymbols(newIdx(1:NUM_TARG));
        for x=1:NUM_TARG
            currentSymbolSet(x) = allSymbols(currentSymbolIdx+x-1);
        end
        currentSymbolIdx = currentSymbolIdx + NUM_TARG;
        
        recenteringState = true;
        currentTarg = NUM_TARG+1;
        lastTarget = uint16(0);
        
        lastAcquireTime = clock;
        state = uint8(SymbolStates.STATE_MOVE_ONE);
        moveTimer = setMoveTimeOne;
    end
elseif state == uint8(SymbolStates.STATE_REHEARSE)
    rehearseTimer = rehearseTimer - 1;
    countdownDisplayTimer = rehearseTimer;
    if rehearseTimer<=5000
        %alert user we are about to begin
        %if mod(rehearseTimer, 1000)==0
        %    lastSoundTime = clock;
        %    lastSoundState = uint8(SequenceStates.SOUND_STATE_SUCCESS);
        %end
    end
    if rehearseTimer<=0
        recenteringState = true;
        currentTarg = NUM_TARG+1;
        lastTarget = uint16(0);
        
        lastAcquireTime = clock;
        state = uint8(SymbolStates.STATE_MOVE_TWO);
        moveTimer = setMoveTimeOne;
    end
    
    %if moving during rehearse, play a sound
    if (filteredHeadSpeed > cursorParameters.headSpeedCap) &&((clock - lastHeadSpeedFail)>2000)
        lastSoundTime = clock;
        lastSoundState = uint8(SequenceStates.SOUND_STATE_FAIL);
        lastHeadSpeedFail = clock;
    end
end

%%
%target acquisition detection
if (state == uint8(SymbolStates.STATE_MOVE_ONE)) || (state == uint8(SymbolStates.STATE_MOVE_TWO))
    effectiveRadius = (cursorParameters.targetDiameter + cursorParameters.cursorDiameter)/2;

    targCollisionIdx = uint16(0);
    for x=1:(NUM_TARG+1)
        targDist = single(sqrt(sum((effectorPos - allTargPos(1:2,x)).^2)));
        if (targDist < effectiveRadius) && lastTarget~=x
            targCollisionIdx = x;
        end
    end
    if targCollisionIdx>0
        holdTimer = holdTimer + 1;
    else
        holdTimer = uint16(0);
    end
    if holdTimer > cursorParameters.holdTime
        %target acquired
        holdTimer = uint16(0);
        lastTarget = targCollisionIdx;
        writeToDiscreteTarg = currentTarg;

        %is it the right target?
        if (currentTarg == targCollisionIdx) || (recenteringState && (targCollisionIdx==(NUM_TARG+1)))
            prevTargAcquireTime = clock - lastAcquireTime;
            lastAcquireTime = clock;
        
            lastSoundTime = clock;
            lastSoundState = uint8(SequenceStates.SOUND_STATE_ACQUIRE);
            showFailedTarg = false;
            
            %track acquire time score
            if ~recenteringState
                summedAcquireTime = summedAcquireTime + prevTargAcquireTime;
                numTargetsAcquired = numTargetsAcquired + 1;
            end
            
            %pick new target
            recenteringState = ~recenteringState;
            if recenteringState
                currentTarg = NUM_TARG+1;
            else
                targetSeqIdx = targetSeqIdx + 1;
                if targetSeqIdx>length(targetSeq)
                    targetSeq = uint16(randperm(NUM_TARG));
                    targetSeqIdx = uint16(1);
                end
                currentTarg = targetSeq(targetSeqIdx);
            end
            writeDiscreteData = true;
        elseif ~showFailedTarg
            lastSoundTime = clock;
            lastSoundState = uint8(SequenceStates.SOUND_STATE_FAIL);
            showFailedTarg = true;
            writeFailedTarg = true;
        end
    end
    
    %transition to next state
    moveTimer = moveTimer - 1;
    if moveTimer <= 0
        if (state == uint8(SymbolStates.STATE_MOVE_ONE))
            
            if rehearseSet
                lastHeadSpeedFail = clock; %don't fail right after entering rehearse state
                state = uint8(SymbolStates.STATE_REHEARSE);
                rehearseTimer = setRehearseTime;
            else
                state = uint8(SymbolStates.STATE_MOVE_TWO);
                moveTimer = setMoveTimeTwo;
            end
            
            %toggle between rehearsing and not rehearsing
            if cursorParameters.symbolVMRMode==1
                rehearseSet = false;
            else
                rehearseSet = ~rehearseSet;
            end
            
        elseif (state == uint8(SymbolStates.STATE_MOVE_TWO))
            numSetsComplete = numSetsComplete + 1;
            state = uint8(SymbolStates.STATE_READY);
            readyTimer = setGetReadyTime;
        end
    end
end

%% PACK DATA FOR UDP OUTPUT (filelogger continuous)
taskOutput.continuous = packFileLoggerFormatAndData('continuous', ...
    TASK_NAME, VERSION_ID, ...
    'clock', clock, ...
    'pause', pauseTriggered, ...
    'xpcRequestClock', behaviorRequestClock, ...
    'peripheralTimestamp', peripheralTimestamp, ...
    'state', state, ...
    'inputType', inputType, ...
    'windowsPacketSize', behaviorPacket.windowsPacketSize, ...
    'windowsMousePosition', behaviorPacket.windowsMousePosition, ...
    'windowsTimestamp', behaviorPacket.windowsTimestamp, ...
    'windowsPC1GazePoint', behaviorPacket.windowsPC1GazePoint, ...
    'windowsPC1GazePointValid', behaviorPacket.windowsPC1GazeValid, ...
    'windowsPC1HeadRot', behaviorPacket.windowsPC1HeadRot, ...
    'windowsPC1HeadRotValid', behaviorPacket.windowsPC1HeadRotValid, ...
    'windowsPC1Timestamp', behaviorPacket.windowsPC1Timestamp, ...
    'pc1MouseInControlMode',cursorParameters.pc1MouseInControlMode, ...
    'xpcScreenUpdateClock',vizPacket.xpcScreenUpdateClock,...
    'pc1MousePos',behaviorPacket.pc1MousePos(1:2).*single([1080; -1080]), ...
    'cursorPosition', single(effectorPos), ...
    'cursorVelocity', single(effectorVel), ...
    'lastTarget', lastTarget, ...
    'taskAgnosticVel', single(effectorVel), ...
    'xk', single(taskOutput.xk),...
    'holdTimer', holdTimer, ...   
    'behaviorPacketSize', behaviorPacket.packetSize, ...
    'xpcTET', single(xpcTET), ...
    'showFailedTarg', showFailedTarg, ...
    'gain', cursorParameters.gain, ...  % not locked  
    'powerGain', cursorParameters.powerGain, ...
    'powerGainUnityCrossing', cursorParameters.powerGain, ...
    'xkModBiasEst', single(xkModBiasEst), ... %the bias estimate coming from the bias killer that acts on xkMod (after nonlinear gain)
    'cognitiveVMRMode', cursorParameters.symbolVMRMode, ...
    'symbolVMRRot', cursorParameters.symbolVMRRot ...    
);

%% SEND DISCRETE DATA TO FILELOGGER
workspaceAll = [cursorParameters.workspaceX; 
    cursorParameters.workspaceY;];

taskOutput.discrete = packFileLoggerFormatAndData('discrete', ...
    TASK_NAME, VERSION_ID, ...
    'clock', clock,...
    'blockNumber', stateParameters.blockNumber,...
    'taskType', cursorParameters.taskType, ...
    'cursorDiameter', single( cursorParameters.cursorDiameter ), ...
    'targetDiameter', single( cursorParameters.targetDiameter ), ...
    'targetSeq', targetSeq, ...
    'acqTimeScore', single(summedAcquireTime)/single(numTargetsAcquired), ...
    'isCenterTarget', ~recenteringState, ...
    'targPosAll', allTargPos(1:2, 1:(NUM_TARG+1)), ...
    'selectedTarget', lastTarget, ...
    'currentTarget', writeToDiscreteTarg, ...
    'holdTime', cursorParameters.holdTime, ...
    'numSetsComplete', numSetsComplete, ...
    'inputType', inputType, ...
    'workspace', workspaceAll, ...    
    'outputType', outputType, ...
    'xk2EffectorPosInds', uint8(effectorPosInds), ...  
    'xk2EffectorVelInds', uint8(effectorVelInds), ...
    'state', state, ...
    'failed', writeFailedTarg, ...
    'isRehearsed', rehearseSet, ...
    'rehearseTime', setRehearseTime, ...
    'currentSymbolSet', currentSymbolSet(1:(NUM_TARG)), ...
    'acqTime', prevTargAcquireTime ...
);

if writeDiscreteData && writeFailedTarg
    writeFailedTarg = false;
end
%% SEND DATA OUT TO VIZ
taskOutput.screen = packFileLoggerFormatAndData('screen', ...
    TASK_NAME, VERSION_ID, ...
    'clock', clock,...
    'blockNumber', stateParameters.blockNumber,...
    'state',state, ...
    'countdownTimer',countdownDisplayTimer, ...
    'acqTimeScore', single(summedAcquireTime)/single(numTargetsAcquired), ...
    'cursorPosition', single(effectorPos), ...
    'cursorColors', cursorColors,...
    'cursorDiameter', cursorParameters.cursorDiameter, ...
    'targetDiameter', cursorParameters.targetDiameter, ...
    'inputType', inputType, ...
    'taskType', cursorParameters.taskType,...
    'numTargets',NUM_TARG+1,...
    'outputType', outputType, ...
    'targetSeq', targetSeq, ...
    'currentTarget', currentTarg, ...
    'lastTarget', lastTarget, ...
    'targPosAll', allTargPos(1:2, 1:(NUM_TARG+1)), ...
    'showFailedTarg', showFailedTarg, ...
    'recentering', recenteringState, ...
    'currentSymbolSet', currentSymbolSet(1:NUM_TARG), ...
    'headMousePos',behaviorPacket.windowsMousePosition(1:2).*single([1080; -1080]), ...
    'pc1MouseInControlMode',cursorParameters.pc1MouseInControlMode, ...
    'cognitiveVMRMode', cursorParameters.symbolVMRMode, ...
    'symbolVMRRot', cursorParameters.symbolVMRRot ...
);

%% SEND DATA OUT TO SOUND
taskOutput.sound = packFileLoggerFormatAndData('screen', ...
    TASK_NAME, VERSION_ID, ...
    'clock', clock,...
    'vizState',state,...
    'lastSoundTime',lastSoundTime,...
    'lastSoundState',lastSoundState...
    ); 

%% SET SEND FLAGS FOR NETWORK OUTPUTS
if(clock < INIT_TIME)
    taskOutput.discrete.data.send = false;
    taskOutput.continuous.data.send = false;
    taskOutput.screen.data.send = false;
    taskOutput.sound.data.send = false;
    
    if(mod(clock, 10)==0)
        taskOutput.sendFormat = true;
    else
        taskOutput.sendFormat = false;
    end
else
    taskOutput.discrete.data.send = writeDiscreteData;
    taskOutput.continuous.data.send = writeContinuousData;
    taskOutput.screen.data.send = true;
    taskOutput.sound.data.send = true;
    taskOutput.sendFormat = false;
    taskOutput.inputType = inputType;
end
taskOutput.wiaCode = uint16(0);
taskOutput.speedCode = uint16(0);
taskOutput.paused = pauseTriggered;

end

function vizPacket = parseVizPacket(packetData)
    vizPacket.xpcScreenUpdateClock = typecast(packetData(28+[1:4]), 'uint32');
end

function vizPacket = initVizPacket()
    vizPacket.xpcScreenUpdateClock = uint32(0);
end
